simulink model "CryoDetFP"  (R2015b)
settings: Solver=ode45  SolverMode=SingleTasking  StartTime=0.0  StopTime=10e-5  MaxStep=1e-9  RelTol=1e-3
values from neighbouring files (symbols this model uses):
  Fclk = Fadc/2    (= 185000000)    [setupCryoFPGA.m]    (also in setupCryoNew.m)
  freqBusAddrBits = 4    [setupCryoNew.m]
  noise = ifft(exp(2i*pi*rand(1, noiseLen)) .* fft(fir1(noiseLen-1, noiseBW/Fclk*noiseSteps)))    [setupCryoFPGA.m]    (also in setupCryoNew.m = exp(2i*pi*rand(1, noiseLen)))
  noiseLen = 128    [setupCryoFPGA.m]    (also in setupCryoNew.m)
  noiseSteps = 32    [setupCryoFPGA.m]    (also in setupCryoNew.m)
  notch = tf( [1 a*wNotch/Q wNotch^2], [1 wNotch/Q wNotch^2])    [setupCryoNew.m]
  notch2 = tf( [1 a*wNotch/Q wNotch^2], [1 wNotch/Q wNotch^2])    [setupCryoNew.m]
  Tclk = 1/Fclk    (= 5.40540540541e-09)    [setupCryoFPGA.m]    (also in setupCryoNew.m)
undefined symbols (not defined in the file or in its folder): AXI4, Lite, notch3, notch4, xlipgetpartsetting
libraries: xbsIndex_r4 x1085
(part 3 of 8)

== system CryoDetFP/DspCore/AdcDac 0/twelveLineUDC 0 ==
  In1 : Inport
  BDC scope : Scope  NumInputPorts=2
  Constant : xbsIndex_r4/Constant  const=0  gui_display_data_type=Fixed-point  arith_type=Unsigned  n_bits=4  bin_pt=0  preci_type=Single  exp_width=8  frac_width=24  explicit_period=off  period=1  equ=P=C  opselect=C  inp2=PCIN>>17  opr=+  inp1=P  carry=CIN  dbl_ovrd=off  block_type=constant
  Constant1 : xbsIndex_r4/Constant  const=1  gui_display_data_type=Fixed-point  arith_type=Unsigned  n_bits=4  bin_pt=0  preci_type=Single  exp_width=8  frac_width=24  explicit_period=off  period=1  equ=P=C  opselect=C  inp2=PCIN>>17  opr=+  inp1=P  carry=CIN  dbl_ovrd=off  block_type=constant
  Constant10 : xbsIndex_r4/Constant  const=10  gui_display_data_type=Fixed-point  arith_type=Unsigned  n_bits=4  bin_pt=0  preci_type=Single  exp_width=8  frac_width=24  explicit_period=off  period=1  equ=P=C  opselect=C  inp2=PCIN>>17  opr=+  inp1=P  carry=CIN  dbl_ovrd=off  block_type=constant
  Constant11 : xbsIndex_r4/Constant  const=11  gui_display_data_type=Fixed-point  arith_type=Unsigned  n_bits=4  bin_pt=0  preci_type=Single  exp_width=8  frac_width=24  explicit_period=off  period=1  equ=P=C  opselect=C  inp2=PCIN>>17  opr=+  inp1=P  carry=CIN  dbl_ovrd=off  block_type=constant
  Constant12 : xbsIndex_r4/Constant  const=15  gui_display_data_type=Fixed-point  arith_type=Unsigned  n_bits=4  bin_pt=0  preci_type=Single  exp_width=8  frac_width=24  explicit_period=off  period=1  equ=P=C  opselect=C  inp2=PCIN>>17  opr=+  inp1=P  carry=CIN  dbl_ovrd=off  block_type=constant
  Constant2 : xbsIndex_r4/Constant  const=2  gui_display_data_type=Fixed-point  arith_type=Unsigned  n_bits=4  bin_pt=0  preci_type=Single  exp_width=8  frac_width=24  explicit_period=off  period=1  equ=P=C  opselect=C  inp2=PCIN>>17  opr=+  inp1=P  carry=CIN  dbl_ovrd=off  block_type=constant
  Constant3 : xbsIndex_r4/Constant  const=3  gui_display_data_type=Fixed-point  arith_type=Unsigned  n_bits=4  bin_pt=0  preci_type=Single  exp_width=8  frac_width=24  explicit_period=off  period=1  equ=P=C  opselect=C  inp2=PCIN>>17  opr=+  inp1=P  carry=CIN  dbl_ovrd=off  block_type=constant
  Constant4 : xbsIndex_r4/Constant  const=4  gui_display_data_type=Fixed-point  arith_type=Unsigned  n_bits=4  bin_pt=0  preci_type=Single  exp_width=8  frac_width=24  explicit_period=off  period=1  equ=P=C  opselect=C  inp2=PCIN>>17  opr=+  inp1=P  carry=CIN  dbl_ovrd=off  block_type=constant
  Constant5 : xbsIndex_r4/Constant  const=5  gui_display_data_type=Fixed-point  arith_type=Unsigned  n_bits=4  bin_pt=0  preci_type=Single  exp_width=8  frac_width=24  explicit_period=off  period=1  equ=P=C  opselect=C  inp2=PCIN>>17  opr=+  inp1=P  carry=CIN  dbl_ovrd=off  block_type=constant
  Constant6 : xbsIndex_r4/Constant  const=6  gui_display_data_type=Fixed-point  arith_type=Unsigned  n_bits=4  bin_pt=0  preci_type=Single  exp_width=8  frac_width=24  explicit_period=off  period=1  equ=P=C  opselect=C  inp2=PCIN>>17  opr=+  inp1=P  carry=CIN  dbl_ovrd=off  block_type=constant
  Constant7 : xbsIndex_r4/Constant  const=7  gui_display_data_type=Fixed-point  arith_type=Unsigned  n_bits=4  bin_pt=0  preci_type=Single  exp_width=8  frac_width=24  explicit_period=off  period=1  equ=P=C  opselect=C  inp2=PCIN>>17  opr=+  inp1=P  carry=CIN  dbl_ovrd=off  block_type=constant
  Constant8 : xbsIndex_r4/Constant  const=8  gui_display_data_type=Fixed-point  arith_type=Unsigned  n_bits=4  bin_pt=0  preci_type=Single  exp_width=8  frac_width=24  explicit_period=off  period=1  equ=P=C  opselect=C  inp2=PCIN>>17  opr=+  inp1=P  carry=CIN  dbl_ovrd=off  block_type=constant
  Constant9 : xbsIndex_r4/Constant  const=9  gui_display_data_type=Fixed-point  arith_type=Unsigned  n_bits=4  bin_pt=0  preci_type=Single  exp_width=8  frac_width=24  explicit_period=off  period=1  equ=P=C  opselect=C  inp2=PCIN>>17  opr=+  inp1=P  carry=CIN  dbl_ovrd=off  block_type=constant
  Counter : xbsIndex_r4/Counter  cnt_type=Count Limited  cnt_to=15  operation=Up  start_count=0  cnt_by_val=1  arith_type=Unsigned  n_bits=4  bin_pt=0  load_pin=off  rst=on  en=on  explicit_period=off  period=Tclk  use_behavioral_HDL=off  implementation=Fabric  dbl_ovrd=off  block_type=counter
  DAC Sum : Subsystem
  Delay : xbsIndex_r4/Delay  rst=off  infoeditControl=Selection of Reset will increase slice count due to use of real FFs and instead of SRLs  en=off  latency=6  reg_retiming=off  dbl_ovrd=off  block_type=delay
  Demux : Demux
  Gateway Out{1,7..10,23} (6 alike) : xbsIndex_r4/Gateway Out  inherit_from_input=off  hdl_port=off  rows=1  columns=1  UseAsDAC=off  DACChannel='1'  interface=None  automatic_assignment=on  address_offset=hex2dec('00')  intf_name=''  intf_description=''  timing_constraint=None  locs_specified=off  LOCs={}  io_standard={}  block_type=gatewayout
  Mux12X4 : Subsystem
  Mux6 : Mux  Inputs=2
  Mux7 : Mux  Inputs=2
  Relational : xbsIndex_r4/Relational  mode=a!=b  op_type=Bool  en=off  latency=0  dbl_ovrd=off  block_type=relational
  SBdemod : Subsystem
  Toolbar : xbsIndex_r4/Toolbar  func=xltoolbar  block_type=toolbar
      settings: infoedit=Toolbar
  oneLineUpDown0 : Subsystem
  oneLineUpDown1 : Subsystem
  oneLineUpDown10 : Subsystem
  oneLineUpDown11 : Subsystem
  oneLineUpDown2 : Subsystem
  oneLineUpDown3 : Subsystem
  oneLineUpDown4 : Subsystem
  oneLineUpDown5 : Subsystem
  oneLineUpDown6 : Subsystem
  oneLineUpDown7 : Subsystem
  oneLineUpDown8 : Subsystem
  oneLineUpDown9 : Subsystem
  synch scope : Scope  NumInputPorts=2
  toDAC : Outport
  demodulated : Outport  Port=2
  wires:
  [fpgaReset] -> Counter/1, Delay/1
  oneLineUpDown7/1(Out1) -> Mux12X4/8(line7)
  oneLineUpDown6/1(Out1) -> Mux12X4/7(line6)
  oneLineUpDown5/1(Out1) -> Mux12X4/6(line5)
  oneLineUpDown4/1(Out1) -> Mux12X4/5(line4)
  oneLineUpDown3/1(Out1) -> Mux12X4/4(line3)
  oneLineUpDown2/1(Out1) -> Mux12X4/3(line2)
  Mux12X4/1(Out1) -> SBdemod/1(In1)
  oneLineUpDown1/1(Out1) -> Mux12X4/2(line1)
  oneLineUpDown0/1(Out1) -> Mux12X4/1(line0)
  oneLineUpDown8/1(Out1) -> Mux12X4/9(line8)
  oneLineUpDown9/1(Out1) -> Mux12X4/10(line9)
  oneLineUpDown10/1(Out1) -> Mux12X4/11(line10)
  oneLineUpDown11/1(Out1) -> Mux12X4/12(line11)
  oneLineUpDown11/2(toDAC) -> DAC Sum/12(In12)
  oneLineUpDown10/2(toDAC) -> DAC Sum/11(In11)
  oneLineUpDown9/2(toDAC) -> DAC Sum/10(In10)
  oneLineUpDown8/2(toDAC) -> DAC Sum/9(In9)
  oneLineUpDown7/2(toDAC) -> DAC Sum/8(In8)
  oneLineUpDown6/2(toDAC) -> DAC Sum/7(In7)
  oneLineUpDown5/2(toDAC) -> DAC Sum/6(In6)
  oneLineUpDown4/2(toDAC) -> DAC Sum/5(In5)
  oneLineUpDown3/2(toDAC) -> DAC Sum/4(In4)
  oneLineUpDown2/2(toDAC) -> DAC Sum/3(In3)
  oneLineUpDown1/2(toDAC) -> DAC Sum/2(In2)
  oneLineUpDown0/2(toDAC) -> DAC Sum/1(In1)
  DAC Sum/1(Out1) -> toDAC/1
  SBdemod/1(AllComponents) -> demodulated/1
  Gateway Out10/1 -> Mux7/2
  Gateway Out9/1 -> Mux7/1
  Gateway Out8/1 -> Mux6/2
  Gateway Out7/1 -> Mux6/1
  Mux6/1 -> BDC scope/1
  Mux7/1 -> BDC scope/2
  Demux/1 -> Gateway Out7/1
  Demux/4 -> Gateway Out10/1
  Demux/3 -> Gateway Out9/1
  Demux/2 -> Gateway Out8/1
  Delay/1 -> Mux12X4/13(synch)
  Constant/1 -> oneLineUpDown0/2(addrIn)
  Constant1/1 -> oneLineUpDown1/2(addrIn)
  Constant2/1 -> oneLineUpDown2/2(addrIn)
  Constant3/1 -> oneLineUpDown3/2(addrIn)
  Constant4/1 -> oneLineUpDown4/2(addrIn)
  Constant5/1 -> oneLineUpDown5/2(addrIn)
  Constant6/1 -> oneLineUpDown6/2(addrIn)
  Constant7/1 -> oneLineUpDown7/2(addrIn)
  Constant8/1 -> oneLineUpDown8/2(addrIn)
  Constant9/1 -> oneLineUpDown9/2(addrIn)
  Constant10/1 -> oneLineUpDown10/2(addrIn)
  Constant11/1 -> oneLineUpDown11/2(addrIn)
  In1/1 -> oneLineUpDown6/1(In), oneLineUpDown8/1(In), oneLineUpDown9/1(In), oneLineUpDown10/1(In), oneLineUpDown11/1(In), oneLineUpDown7/1(In), Demux/1, oneLineUpDown5/1(In), oneLineUpDown4/1(In), oneLineUpDown3/1(In), oneLineUpDown2/1(In), oneLineUpDown1/1(In), oneLineUpDown0/1(In)
  Counter/1 -> Gateway Out23/1, Relational/2, oneLineUpDown2/3(synchIn), oneLineUpDown3/3(synchIn), oneLineUpDown4/3(synchIn), oneLineUpDown5/3(synchIn), oneLineUpDown6/3(synchIn), oneLineUpDown7/3(synchIn), oneLineUpDown8/3(synchIn), oneLineUpDown10/3(synchIn), oneLineUpDown11/3(synchIn), oneLineUpDown9/3(synchIn), oneLineUpDown1/3(synchIn), oneLineUpDown0/3(synchIn)
  Gateway Out23/1 -> synch scope/1
  Gateway Out1/1 -> synch scope/2
  Relational/1 -> Gateway Out1/1, Counter/2
  Constant12/1 -> Relational/1

== system CryoDetFP/DspCore/AdcDac 0/twelveLineUDC 1 ==
  note: Null for now, eventually copy twelveLineUDC 0
      | when we need more than 12 lines per ADC channel
  In1 : Inport
  Out1 : Outport
  wires:
  In1/1 -> Out1/1

== system CryoDetFP/DspCore/AdcDac 0/SBmodulator/Phase Modulator ==
  Iin : Inport
  Qin : Inport  Port=2
  Ipm : Inport  Port=3
  Qpm : Inport  Port=4
  AddSub : xbsIndex_r4/AddSub  mode=Subtraction  use_carryin=off  use_carryout=off  en=off  latency=1  precision=User Defined  arith_type="Signed  (2's comp)"  n_bits=16  bin_pt=15  quantization=Truncate  overflow=Wrap  use_behavioral_HDL=off  hw_selection=Fabric  pipelined=off  dbl_ovrd=off  block_type=addsub
  AddSub1 : xbsIndex_r4/AddSub  mode=Addition  use_carryin=off  use_carryout=off  en=off  latency=1  precision=User Defined  arith_type="Signed  (2's comp)"  n_bits=16  bin_pt=15  quantization=Truncate  overflow=Wrap  use_behavioral_HDL=off  hw_selection=Fabric  pipelined=off  dbl_ovrd=off  block_type=addsub
  Mult{1..4} (4 alike) : xbsIndex_r4/Mult  precision=User Defined  arith_type="Signed  (2's comp)"  n_bits=16  bin_pt=15  quantization=Truncate  overflow=Wrap  en=off  latency=3  use_behavioral_HDL=off  opt=Speed  use_embedded=on  optimum_pipeline=off  pipeline=on  dbl_ovrd=off  use_rpm=on  placement_style=Triangular  block_type=mult
  Iout : Outport
  Qout : Outport  Port=2
  wires:
  Iin/1 -> Mult4/1, Mult2/1
  Qin/1 -> Mult1/1, Mult3/1
  Ipm/1 -> Mult2/2, Mult1/2
  Qpm/1 -> Mult3/2, Mult4/2
  Mult2/1 -> AddSub/1
  Mult3/1 -> AddSub/2
  Mult1/1 -> AddSub1/1
  Mult4/1 -> AddSub1/2
  AddSub/1 -> Iout/1
  AddSub1/1 -> Qout/1

== system CryoDetFP/DspCore/AdcDac 0/dF/CplxProd ==
  tvalidIn : Inport
  Im_A : Inport  Port=2
  Re_A : Inport  Port=3
  Im_B : Inport  Port=4
  Re_B : Inport  Port=5
  AddSub : xbsIndex_r4/AddSub  mode=Subtraction  use_carryin=off  use_carryout=off  en=off  latency=3  precision=Full  arith_type=Unsigned  n_bits=16  bin_pt=14  quantization=Truncate  overflow=Wrap  use_behavioral_HDL=off  hw_selection=Fabric  pipelined=off  dbl_ovrd=off  block_type=addsub
  AddSub1 : xbsIndex_r4/AddSub  mode=Addition  use_carryin=off  use_carryout=off  en=off  latency=3  precision=Full  arith_type=Unsigned  n_bits=16  bin_pt=14  quantization=Truncate  overflow=Wrap  use_behavioral_HDL=off  hw_selection=Fabric  pipelined=off  dbl_ovrd=off  block_type=addsub
  Delay : xbsIndex_r4/Delay  rst=off  infoeditControl=Selection of Reset will increase slice count due to use of real FFs and instead of SRLs  en=off  latency=3  reg_retiming=off  dbl_ovrd=off  block_type=delay
  Delay1 : xbsIndex_r4/Delay  rst=off  infoeditControl=Selection of Reset will increase slice count due to use of real FFs and instead of SRLs  en=off  latency=3  reg_retiming=off  dbl_ovrd=off  block_type=delay
  Mult{,1..3} (4 alike) : xbsIndex_r4/Mult  precision=Full  arith_type="Signed  (2's comp)"  n_bits=16  bin_pt=14  quantization=Truncate  overflow=Wrap  en=off  latency=3  use_behavioral_HDL=off  opt=Speed  use_embedded=on  optimum_pipeline=off  pipeline=on  dbl_ovrd=off  use_rpm=on  placement_style=Triangular  block_type=mult
  tvalidOut : Outport
  Im_Out : Outport  Port=2
  Re_Out : Outport  Port=3
  wires:
  Delay/1 -> Delay1/1
  Mult2/1 -> AddSub1/1
  Mult/1 -> AddSub/1
  Mult1/1 -> AddSub/2
  Mult3/1 -> AddSub1/2
  Re_A/1 -> Mult3/1, Mult/1
  Im_A/1 -> Mult2/1, Mult1/1
  tvalidIn/1 -> Delay/1
  Im_B/1 -> Mult1/2, Mult3/2
  Re_B/1 -> Mult/2, Mult2/2
  Delay1/1 -> tvalidOut/1
  AddSub/1 -> Re_Out/1
  AddSub1/1 -> Im_Out/1

== system CryoDetFP/DspCore/AdcDac 0/dF/CplxProd1 ==
  tvalidIn : Inport
  Im_A : Inport  Port=2
  Re_A : Inport  Port=3
  Im_B : Inport  Port=4
  Re_B : Inport  Port=5
  AddSub : xbsIndex_r4/AddSub  mode=Subtraction  use_carryin=off  use_carryout=off  en=off  latency=3  precision=Full  arith_type=Unsigned  n_bits=16  bin_pt=14  quantization=Truncate  overflow=Wrap  use_behavioral_HDL=off  hw_selection=Fabric  pipelined=off  dbl_ovrd=off  block_type=addsub
  AddSub1 : xbsIndex_r4/AddSub  mode=Addition  use_carryin=off  use_carryout=off  en=off  latency=3  precision=Full  arith_type=Unsigned  n_bits=16  bin_pt=14  quantization=Truncate  overflow=Wrap  use_behavioral_HDL=off  hw_selection=Fabric  pipelined=off  dbl_ovrd=off  block_type=addsub
  Delay : xbsIndex_r4/Delay  rst=off  infoeditControl=Selection of Reset will increase slice count due to use of real FFs and instead of SRLs  en=off  latency=3  reg_retiming=off  dbl_ovrd=off  block_type=delay
  Delay1 : xbsIndex_r4/Delay  rst=off  infoeditControl=Selection of Reset will increase slice count due to use of real FFs and instead of SRLs  en=off  latency=3  reg_retiming=off  dbl_ovrd=off  block_type=delay
  Mult{,1..3} (4 alike) : xbsIndex_r4/Mult  precision=Full  arith_type="Signed  (2's comp)"  n_bits=16  bin_pt=14  quantization=Truncate  overflow=Wrap  en=off  latency=3  use_behavioral_HDL=off  opt=Speed  use_embedded=on  optimum_pipeline=off  pipeline=on  dbl_ovrd=off  use_rpm=on  placement_style=Triangular  block_type=mult
  tvalidOut : Outport
  Im_Out : Outport  Port=2
  Re_Out : Outport  Port=3
  wires:
  Delay/1 -> Delay1/1
  Mult2/1 -> AddSub1/1
  Mult/1 -> AddSub/1
  Mult1/1 -> AddSub/2
  Mult3/1 -> AddSub1/2
  Re_A/1 -> Mult3/1, Mult/1
  Im_A/1 -> Mult2/1, Mult1/1
  tvalidIn/1 -> Delay/1
  Im_B/1 -> Mult1/2, Mult3/2
  Re_B/1 -> Mult/2, Mult2/2
  Delay1/1 -> tvalidOut/1
  AddSub/1 -> Re_Out/1
  AddSub1/1 -> Im_Out/1

== system CryoDetFP/DspCore/AdcDac 0/dF/etaRAM ==
  note: 4 May 2016 Now floating point
  readAddr : Inport
  "etaBusIn " : Inport  Port=2
  Bus Selector : BusSelector  OutputSignals=channel,etaQ,etaI
  Concat : xbsIndex_r4/Concat  num_inputs=2  dbl_ovrd=off  block_type=concat
  Dual Port RAM : xbsIndex_r4/Dual Port RAM  depth=2^freqBusAddrBits  initVector=0  distributed_mem=Block RAM  init_a=0  init_b=0  rst_a=off  rst_b=off  en_a=off  en_b=off  latency=2  write_mode_A=Read Before Write  write_mode_B=Read After Write  optimize=Area  dbl_ovrd=off  block_type=dpram
  Gateway Out{1..3,13,26,29} (6 alike) : xbsIndex_r4/Gateway Out  inherit_from_input=off  hdl_port=off  rows=1  columns=1  UseAsDAC=off  DACChannel='1'  interface=None  automatic_assignment=on  address_offset=hex2dec('00')  intf_name=''  intf_description=''  timing_constraint=None  locs_specified=off  LOCs={}  io_standard={}  block_type=gatewayout
  Mux1 : Mux  Inputs=2
  Mux13 : Mux  Inputs=2
  Mux7 : Mux  Inputs=2
  Reinterpret : xbsIndex_r4/Reinterpret  force_arith_type=on  arith_type=Unsigned  force_bin_pt=on  bin_pt=0  block_type=reinterpret
  Reinterpret1 : xbsIndex_r4/Reinterpret  force_arith_type=on  arith_type=Unsigned  force_bin_pt=on  bin_pt=0  block_type=reinterpret
  Reinterpret2 : xbsIndex_r4/Reinterpret  force_arith_type=on  arith_type=Floating-point  force_bin_pt=on  bin_pt=24  block_type=reinterpret
  Reinterpret3 : xbsIndex_r4/Reinterpret  force_arith_type=on  arith_type=Floating-point  force_bin_pt=on  bin_pt=24  block_type=reinterpret
  Slice : xbsIndex_r4/Slice  nbits=32  boolean_output=off  mode=Upper Bit Location + Width  bit1=0  base1=MSB of Input  bit0=0  base0=LSB of Input  dbl_ovrd=off  block_type=slice
  Slice1 : xbsIndex_r4/Slice  nbits=32  boolean_output=off  mode=Lower Bit Location + Width  bit1=0  base1=MSB of Input  bit0=0  base0=LSB of Input  dbl_ovrd=off  block_type=slice
  Terminator3 : Terminator
  eta ram in out : Scope  NumInputPorts=3
  read : xbsIndex_r4/Constant  const=0  gui_display_data_type=Boolean  arith_type=Boolean  n_bits=16  bin_pt=14  preci_type=Single  exp_width=8  frac_width=24  explicit_period=off  period=1  equ=P=C  opselect=C  inp2=PCIN>>17  opr=+  inp1=P  carry=CIN  dbl_ovrd=off  block_type=constant
  write : xbsIndex_r4/Constant  const=1.0  gui_display_data_type=Boolean  arith_type=Boolean  n_bits=16  bin_pt=14  preci_type=Single  exp_width=8  frac_width=24  explicit_period=off  period=1  equ=P=C  opselect=C  inp2=PCIN>>17  opr=+  inp1=P  carry=CIN  dbl_ovrd=off  block_type=constant
  etaQ : Outport
  etaI : Outport  Port=2
  wires:
  read/1 -> Dual Port RAM/6
  Bus Selector/1 -> Gateway Out26/1, Dual Port RAM/1  "<channel>"
  write/1 -> Dual Port RAM/3
  Dual Port RAM/2 -> Slice1/1, Slice/1
  Dual Port RAM/1 -> Terminator3/1
  "etaBusIn "/1 -> Bus Selector/1
  Bus Selector/2 -> Gateway Out2/1, Reinterpret/1  "<etaQ>"
  Bus Selector/3 -> Gateway Out29/1, Reinterpret1/1  "<etaI>"
  Reinterpret1/1 -> Concat/2
  Reinterpret/1 -> Concat/1
  Concat/1 -> Dual Port RAM/2, Dual Port RAM/5
  Slice/1 -> Reinterpret2/1
  Slice1/1 -> Reinterpret3/1
  Reinterpret2/1 -> Gateway Out1/1, etaQ/1
  Reinterpret3/1 -> Gateway Out3/1, etaI/1
  Gateway Out29/1 -> Mux13/1
  Mux13/1 -> eta ram in out/2
  Gateway Out13/1 -> Mux7/2
  Gateway Out26/1 -> Mux7/1
  Mux7/1 -> eta ram in out/1
  Gateway Out2/1 -> Mux13/2
  readAddr/1 -> Gateway Out13/1, Dual Port RAM/4
  Gateway Out3/1 -> Mux1/1
  Mux1/1 -> eta ram in out/3
  Gateway Out1/1 -> Mux1/2

== system CryoDetFP/DspCore/AdcDac 0/eta/Complex Divide ==
  note: Complex multiplier has latency 6
  a_tvalid : Inport
  A_Q : Inport  Port=2
  A_I : Inport  Port=3
  b_tvalid : Inport  Port=4
  B_Q : Inport  Port=5
  B_I : Inport  Port=6
  AddSub : xbsIndex_r4/AddSub  mode=Addition  use_carryin=off  use_carryout=off  en=off  latency=3  precision=Full  arith_type="Signed  (2's comp)"  n_bits=48  bin_pt=44  quantization=Truncate  overflow=Flag as error  use_behavioral_HDL=on  hw_selection=Fabric  pipelined=off  dbl_ovrd=off  block_type=addsub
  CMult : xbsIndex_r4/CMult  const=-1  gui_display_data_type=Floating-point  const_n_bits=16  const_bin_pt=15  float_type=Single  exp_bits=8  fraction_bits=24  en=off  latency=1  precision=Full  arith_type="Signed  (2's comp)"  n_bits=32  bin_pt=30  quantization=Truncate  overflow=Wrap  use_behavioral_HDL=off  mem_type=Distributed RAM  pipeline=off  dbl_ovrd=off  block_type=cmult
  Constant : xbsIndex_r4/Constant  const=0  gui_display_data_type=Floating-point  arith_type=Floating-point  n_bits=63  bin_pt=15  preci_type=Single  exp_width=8  frac_width=24  explicit_period=off  period=1  equ=P=C  opselect=C  inp2=PCIN>>17  opr=+  inp1=P  carry=CIN  dbl_ovrd=off  block_type=constant
  Cplx Div 2 : Scope  NumInputPorts=3
  CplxProd : Subsystem
  Cpx Div : Scope  NumInputPorts=4
  Delay{,1..2,5} (4 alike) : xbsIndex_r4/Delay  rst=off  infoeditControl=Selection of Reset will increase slice count due to use of real FFs and instead of SRLs  en=off  latency=1  reg_retiming=on  dbl_ovrd=off  block_type=delay
  Delay3 : xbsIndex_r4/Delay  rst=off  infoeditControl=Selection of Reset will increase slice count due to use of real FFs and instead of SRLs  en=off  latency=8  reg_retiming=on  dbl_ovrd=off  block_type=delay
  Divide : xbsIndex_r4/Divide  flow_control=NonBlocking  axi_optimize_goal=Resources  algorithm_type=Radix2  infoedit1=Specify output fraction-width for Fixed-point division.  fractional_width=24  infoedit2=Specify latency for Floating-point division.  latency=8  rate=1  has_a_tlast=off  has_a_tuser=off  has_b_tlast=off  has_b_tuser=off  en=off  has_result_tready=off  result_tlast_behv=Pass_A_TLAST  has_underflow=on  has_overflow=on  has_invalid_op=on  has_divide_by_zero=on  fpo_op_type=mergeddivide  block_type=divide
      settings: infoedit=Blocking: Wait for data on all inputs, allow back-pressure.<br>NonBlocking: operate every cycle in which all inputs are valid, no back-pressure.
  Divide1 : xbsIndex_r4/Divide  flow_control=NonBlocking  axi_optimize_goal=Resources  algorithm_type=Radix2  infoedit1=Specify output fraction-width for Fixed-point division.  fractional_width=24  infoedit2=Specify latency for Floating-point division.  latency=8  rate=1  has_a_tlast=off  has_a_tuser=off  has_b_tlast=off  has_b_tuser=off  en=off  has_result_tready=off  result_tlast_behv=Pass_A_TLAST  has_underflow=on  has_overflow=on  has_invalid_op=on  has_divide_by_zero=on  fpo_op_type=mergeddivide  block_type=divide
      settings: infoedit=Blocking: Wait for data on all inputs, allow back-pressure.<br>NonBlocking: operate every cycle in which all inputs are valid, no back-pressure.
  Gateway Out{6..17} (12 alike) : xbsIndex_r4/Gateway Out  inherit_from_input=off  hdl_port=off  rows=1  columns=1  UseAsDAC=off  DACChannel='1'  interface=None  automatic_assignment=on  address_offset=hex2dec('00')  intf_name=''  intf_description=''  timing_constraint=None  locs_specified=off  LOCs={}  io_standard={}  block_type=gatewayout
  Mult : xbsIndex_r4/Mult  precision=Full  arith_type="Signed  (2's comp)"  n_bits=48  bin_pt=44  quantization=Truncate  overflow=Flag as error  en=off  latency=4  use_behavioral_HDL=on  opt=Speed  use_embedded=on  optimum_pipeline=on  pipeline=on  dbl_ovrd=off  use_rpm=on  placement_style=Triangular  block_type=mult
  Mult1 : xbsIndex_r4/Mult  precision=Full  arith_type="Signed  (2's comp)"  n_bits=48  bin_pt=44  quantization=Truncate  overflow=Flag as error  en=off  latency=4  use_behavioral_HDL=on  opt=Speed  use_embedded=on  optimum_pipeline=off  pipeline=on  dbl_ovrd=off  use_rpm=on  placement_style=Triangular  block_type=mult
  Mux{1,3..5,8..10} (7 alike) : Mux  Inputs=2
  Mux6 : xbsIndex_r4/Mux  inputs=2  en=off  latency=0  precision=Full  arith_type=Unsigned  n_bits=63  bin_pt=15  quantization=Truncate  overflow=Flag as error  dbl_ovrd=off  block_type=mux
  Mux7 : xbsIndex_r4/Mux  inputs=2  en=off  latency=0  precision=Full  arith_type=Unsigned  n_bits=63  bin_pt=15  quantization=Truncate  overflow=Flag as error  dbl_ovrd=off  block_type=mux
  Terminator5 : Terminator
  tvalidOut : Outport
  Out_Q : Outport  Port=2
  Out_I : Outport  Port=3
  invalid op : Outport  Port=4
  wires:
  a_tvalid/1 -> Gateway Out13/1, Gateway Out12/1, Delay/1
  A_Q/1 -> Delay1/1, Gateway Out14/1
  A_I/1 -> Delay2/1, Gateway Out15/1
  Divide/1 -> Mux7/2
  Mult1/1 -> AddSub/2
  AddSub/1 -> Divide/2, Divide1/2
  Divide1/4 -> Gateway Out11/1, invalid op/1, Mux6/1, Mux7/1
  Mux7/1 -> Gateway Out6/1, Out_Q/1
  Mux6/1 -> Out_I/1, Gateway Out7/1
  Mult/1 -> AddSub/1
  Gateway Out6/1 -> Mux3/1
  Gateway Out7/1 -> Mux3/2
  Gateway Out8/1 -> Mux4/1
  Gateway Out9/1 -> Mux4/2
  Gateway Out10/1 -> Mux5/1
  Gateway Out11/1 -> Mux5/2
  Divide1/1 -> Mux6/2
  Constant/1 -> Mux7/3, Mux6/3
  Delay5/1 -> CplxProd/5(Re_B)
  Delay2/1 -> CplxProd/3(Re_A)
  Delay1/1 -> CplxProd/2(Im_A)
  Delay/1 -> CplxProd/1(tvalidIn)
  B_Q/1 -> Mult1/1, Mult1/2, Gateway Out16/1, CMult/1
  B_I/1 -> Mult/1, Mult/2, Delay5/1, Gateway Out17/1
  CMult/1 -> CplxProd/4(Im_B)
  Gateway Out12/1 -> Mux8/1
  Gateway Out13/1 -> Mux8/2
  Gateway Out14/1 -> Mux9/1
  Gateway Out15/1 -> Mux9/2
  Gateway Out16/1 -> Mux10/1
  Gateway Out17/1 -> Mux10/2
  Mux8/1 -> Cplx Div 2/1
  Mux9/1 -> Cplx Div 2/2
  Mux10/1 -> Cplx Div 2/3
  b_tvalid/1 -> Terminator5/1
  CplxProd/2(Im_Out) -> Divide/1
  CplxProd/1(tvalidOut) -> Mux1/2, Delay3/1
  CplxProd/3(Re_Out) -> Divide1/1
  Divide1/2 -> Gateway Out8/1
  Divide1/3 -> Gateway Out9/1
  Divide1/5 -> Gateway Out10/1
  Mux3/1 -> Cpx Div/2
  Mux4/1 -> Cpx Div/3
  Mux5/1 -> Cpx Div/4
  Delay3/1 -> Mux1/1, tvalidOut/1
  Mux1/1 -> Cpx Div/1

== system CryoDetFP/DspCore/AdcDac 0/eta/CplxProd ==
  tvalidIn : Inport
  Im_A : Inport  Port=2
  Re_A : Inport  Port=3
  Im_B : Inport  Port=4
  Re_B : Inport  Port=5
  AddSub : xbsIndex_r4/AddSub  mode=Subtraction  use_carryin=off  use_carryout=off  en=off  latency=3  precision=Full  arith_type=Unsigned  n_bits=16  bin_pt=14  quantization=Truncate  overflow=Wrap  use_behavioral_HDL=off  hw_selection=Fabric  pipelined=off  dbl_ovrd=off  block_type=addsub
  AddSub1 : xbsIndex_r4/AddSub  mode=Addition  use_carryin=off  use_carryout=off  en=off  latency=3  precision=Full  arith_type=Unsigned  n_bits=16  bin_pt=14  quantization=Truncate  overflow=Wrap  use_behavioral_HDL=off  hw_selection=Fabric  pipelined=off  dbl_ovrd=off  block_type=addsub
  Delay : xbsIndex_r4/Delay  rst=off  infoeditControl=Selection of Reset will increase slice count due to use of real FFs and instead of SRLs  en=off  latency=3  reg_retiming=off  dbl_ovrd=off  block_type=delay
  Delay1 : xbsIndex_r4/Delay  rst=off  infoeditControl=Selection of Reset will increase slice count due to use of real FFs and instead of SRLs  en=off  latency=3  reg_retiming=off  dbl_ovrd=off  block_type=delay
  Mult{,1..3} (4 alike) : xbsIndex_r4/Mult  precision=Full  arith_type="Signed  (2's comp)"  n_bits=16  bin_pt=14  quantization=Truncate  overflow=Wrap  en=off  latency=3  use_behavioral_HDL=off  opt=Speed  use_embedded=on  optimum_pipeline=off  pipeline=on  dbl_ovrd=off  use_rpm=on  placement_style=Triangular  block_type=mult
  tvalidOut : Outport
  Im_Out : Outport  Port=2
  Re_Out : Outport  Port=3
  wires:
  Delay/1 -> Delay1/1
  Mult2/1 -> AddSub1/1
  Mult/1 -> AddSub/1
  Mult1/1 -> AddSub/2
  Mult3/1 -> AddSub1/2
  Re_A/1 -> Mult3/1, Mult/1
  Im_A/1 -> Mult2/1, Mult1/1
  tvalidIn/1 -> Delay/1
  Im_B/1 -> Mult1/2, Mult3/2
  Re_B/1 -> Mult/2, Mult2/2
  Delay1/1 -> tvalidOut/1
  AddSub/1 -> Re_Out/1
  AddSub1/1 -> Im_Out/1

== system CryoDetFP/DspCore/AdcDac 0/eta/CplxProd1 ==
  tvalidIn : Inport
  Im_A : Inport  Port=2
  Re_A : Inport  Port=3
  Im_B : Inport  Port=4
  Re_B : Inport  Port=5
  AddSub : xbsIndex_r4/AddSub  mode=Subtraction  use_carryin=off  use_carryout=off  en=off  latency=3  precision=Full  arith_type=Unsigned  n_bits=16  bin_pt=14  quantization=Truncate  overflow=Wrap  use_behavioral_HDL=off  hw_selection=Fabric  pipelined=off  dbl_ovrd=off  block_type=addsub
  AddSub1 : xbsIndex_r4/AddSub  mode=Addition  use_carryin=off  use_carryout=off  en=off  latency=3  precision=Full  arith_type=Unsigned  n_bits=16  bin_pt=14  quantization=Truncate  overflow=Wrap  use_behavioral_HDL=off  hw_selection=Fabric  pipelined=off  dbl_ovrd=off  block_type=addsub
  Delay : xbsIndex_r4/Delay  rst=off  infoeditControl=Selection of Reset will increase slice count due to use of real FFs and instead of SRLs  en=off  latency=3  reg_retiming=off  dbl_ovrd=off  block_type=delay
  Delay1 : xbsIndex_r4/Delay  rst=off  infoeditControl=Selection of Reset will increase slice count due to use of real FFs and instead of SRLs  en=off  latency=3  reg_retiming=off  dbl_ovrd=off  block_type=delay
  Mult{,1..3} (4 alike) : xbsIndex_r4/Mult  precision=Full  arith_type="Signed  (2's comp)"  n_bits=16  bin_pt=14  quantization=Truncate  overflow=Wrap  en=off  latency=3  use_behavioral_HDL=off  opt=Speed  use_embedded=on  optimum_pipeline=off  pipeline=on  dbl_ovrd=off  use_rpm=on  placement_style=Triangular  block_type=mult
  tvalidOut : Outport
  Im_Out : Outport  Port=2
  Re_Out : Outport  Port=3
  wires:
  Delay/1 -> Delay1/1
  Mult2/1 -> AddSub1/1
  Mult/1 -> AddSub/1
  Mult1/1 -> AddSub/2
  Mult3/1 -> AddSub1/2
  Re_A/1 -> Mult3/1, Mult/1
  Im_A/1 -> Mult2/1, Mult1/1
  tvalidIn/1 -> Delay/1
  Im_B/1 -> Mult1/2, Mult3/2
  Re_B/1 -> Mult/2, Mult2/2
  Delay1/1 -> tvalidOut/1
  AddSub/1 -> Re_Out/1
  AddSub1/1 -> Im_Out/1

== system CryoDetFP/DspCore/AdcDac 0/eta/CplxProd2 ==
  tvalidIn : Inport
  Im_A : Inport  Port=2
  Re_A : Inport  Port=3
  Im_B : Inport  Port=4
  Re_B : Inport  Port=5
  AddSub : xbsIndex_r4/AddSub  mode=Subtraction  use_carryin=off  use_carryout=off  en=off  latency=3  precision=Full  arith_type=Unsigned  n_bits=16  bin_pt=14  quantization=Truncate  overflow=Wrap  use_behavioral_HDL=off  hw_selection=Fabric  pipelined=off  dbl_ovrd=off  block_type=addsub
  AddSub1 : xbsIndex_r4/AddSub  mode=Addition  use_carryin=off  use_carryout=off  en=off  latency=3  precision=Full  arith_type=Unsigned  n_bits=16  bin_pt=14  quantization=Truncate  overflow=Wrap  use_behavioral_HDL=off  hw_selection=Fabric  pipelined=off  dbl_ovrd=off  block_type=addsub
  Delay : xbsIndex_r4/Delay  rst=off  infoeditControl=Selection of Reset will increase slice count due to use of real FFs and instead of SRLs  en=off  latency=3  reg_retiming=off  dbl_ovrd=off  block_type=delay
  Delay1 : xbsIndex_r4/Delay  rst=off  infoeditControl=Selection of Reset will increase slice count due to use of real FFs and instead of SRLs  en=off  latency=3  reg_retiming=off  dbl_ovrd=off  block_type=delay
  Mult{,1..3} (4 alike) : xbsIndex_r4/Mult  precision=Full  arith_type="Signed  (2's comp)"  n_bits=16  bin_pt=14  quantization=Truncate  overflow=Wrap  en=off  latency=3  use_behavioral_HDL=off  opt=Speed  use_embedded=on  optimum_pipeline=off  pipeline=on  dbl_ovrd=off  use_rpm=on  placement_style=Triangular  block_type=mult
  tvalidOut : Outport
  Im_Out : Outport  Port=2
  Re_Out : Outport  Port=3
  wires:
  Delay/1 -> Delay1/1
  Mult2/1 -> AddSub1/1
  Mult/1 -> AddSub/1
  Mult1/1 -> AddSub/2
  Mult3/1 -> AddSub1/2
  Re_A/1 -> Mult3/1, Mult/1
  Im_A/1 -> Mult2/1, Mult1/1
  tvalidIn/1 -> Delay/1
  Im_B/1 -> Mult1/2, Mult3/2
  Re_B/1 -> Mult/2, Mult2/2
  Delay1/1 -> tvalidOut/1
  AddSub/1 -> Re_Out/1
  AddSub1/1 -> Im_Out/1

== system CryoDetFP/DspCore/AdcDac 0/eta/LPF ==
  note: REF channel should not be low-passed!
      | Needs to have same bandwidth as signal channel
      | but latency must match
  note: streaming interface? so complex divide gets data at lower rate?
  note: tvalid
  note: Channel #
  note: Sig+
  note: Sig-
  note: Ref+
  note: Ref
  note: Sig
  note: Ref-
  In1 : Inport
  Bus Creator : BusCreator  Inputs=2
  Bus Creator1 : BusCreator  Inputs=2
  Bus Selector : BusSelector  OutputSignals=chanAndTvalid,signal2
  Bus Selector1 : BusSelector  OutputSignals=channel,valid
  Bus Selector2 : BusSelector  OutputSignals=channel,tvalid
  CIC Compiler 4.0 {1..10} (10 alike) : xbsIndex_r4/CIC Compiler 4.0   filter_type=Decimation  number_of_stages=3  differential_delay=1  number_of_channels=12  sample_rate_changes=Fixed  fixed_or_initial_rate=8  minimum_rate=8  maximum_rate=8  ratespecification=Sample_Period  sampleperiod=1  hardwareoversamplingrate=1  quantization=Truncation  output_data_width=24  use_xtreme_dsp_slice=off  use_streaming_interface=on  has_aclken=off  has_aresetn=on  has_dout_tready=off  trim_axipin_name=on  gui_behaviour=Sysgen_GUI  input_data_width=18  ip_name=CIC Compiler  ip_version=4.0  dsptool_ready=true  wrapper_available=true  port_translation_map={ 'aclken' => 'en', 'aresetn' => 'rst' }  ipcore_xco_need_fpga_part=true  ipcore_verbose=false  block_type=cic_compiler_v4_0
  CIC LPF Scope : Scope  NumInputPorts=6
  CIC LPF input scope : Scope  NumInputPorts=5
  CIC reset : Subsystem
  Constant4 : xbsIndex_r4/Constant  const=10  gui_display_data_type=Fixed-point  arith_type=Unsigned  n_bits=4  bin_pt=0  preci_type=Single  exp_width=8  frac_width=24  explicit_period=off  period=1  equ=P=C  opselect=C  inp2=PCIN>>17  opr=+  inp1=P  carry=CIN  dbl_ovrd=off  block_type=constant
  Demux{,3..6} (5 alike) : Demux  Outputs=2
  Demux1 : Demux  Outputs=6
  Display : Display
  Gateway Out{,1,5..18} (16 alike) : xbsIndex_r4/Gateway Out  inherit_from_input=off  hdl_port=off  rows=1  columns=1  UseAsDAC=off  DACChannel='1'  interface=None  automatic_assignment=on  address_offset=hex2dec('00')  intf_name=''  intf_description=''  timing_constraint=None  locs_specified=off  LOCs={}  io_standard={}  block_type=gatewayout
  LPF chan output : Scope  NumInputPorts=2
  Mux : Mux  Inputs=2
  Mux1 : Mux  Inputs=10
  Mux3 : Mux  Inputs=2
  Mux4 : Mux  Inputs=2
  Scale{,1..9} (10 alike) : xbsIndex_r4/Scale  scale_factor=-9  dbl_ovrd=off  block_type=scale
  Terminator : Terminator
  Out1 : Outport
  wires:
  Demux1/1 -> Terminator/1
  Demux1/2 -> Demux/1
  Demux1/3 -> Demux3/1
  Demux1/5 -> Demux5/1
  Demux1/6 -> Demux6/1
  Bus Selector/2 -> Demux1/1  "<signal2>"
  In1/1 -> Bus Selector/1
  Demux1/4 -> Demux4/1
  Demux/1 -> Gateway Out16/1, CIC Compiler 4.0 3/2
  Demux/2 -> CIC Compiler 4.0 1/2
  Demux3/1 -> CIC Compiler 4.0 2/2
  Demux3/2 -> CIC Compiler 4.0 4/2
  Demux5/1 -> CIC Compiler 4.0 7/2
  Demux5/2 -> CIC Compiler 4.0 8/2
  Demux6/1 -> CIC Compiler 4.0 9/2
  Demux6/2 -> CIC Compiler 4.0 10/2
  Bus Selector1/2 -> CIC Compiler 4.0 3/1, CIC Compiler 4.0 1/1, CIC Compiler 4.0 2/1, CIC Compiler 4.0 4/1, CIC Compiler 4.0 5/1, CIC Compiler 4.0 6/1, CIC Compiler 4.0 7/1, CIC Compiler 4.0 8/1, CIC Compiler 4.0 9/1, CIC Compiler 4.0 10/1  "<valid>"
  Bus Selector1/1 -> Gateway Out15/1, CIC reset/2(Channel), [ChanIn]  "<channel>"
  Bus Selector/1 -> Bus Selector1/1  "<chanAndTvalid>"
  CIC Compiler 4.0 3/3 -> Scale/1
  CIC Compiler 4.0 1/3 -> Scale1/1
  CIC Compiler 4.0 2/3 -> Scale2/1
  CIC Compiler 4.0 4/3 -> Scale3/1
  Demux4/1 -> CIC Compiler 4.0 5/2
  Demux4/2 -> CIC Compiler 4.0 6/2
  CIC Compiler 4.0 7/3 -> Scale4/1
  CIC Compiler 4.0 8/3 -> Scale5/1
  CIC Compiler 4.0 9/3 -> Scale6/1
  CIC Compiler 4.0 10/3 -> Scale7/1
  Mux1/1 -> Bus Creator/2
  Bus Creator/1 -> Out1/1
  Bus Creator1/1 -> Bus Creator/1, Bus Selector2/1
  Scale/1 -> Gateway Out1/1, Mux1/1
  Scale1/1 -> Mux1/2
  Scale2/1 -> Mux1/3
  Scale3/1 -> Mux1/4
  Scale4/1 -> Mux1/7
  Scale5/1 -> Mux1/8
  Scale6/1 -> Mux1/9
  Scale7/1 -> Mux1/10
  CIC Compiler 4.0 7/2 -> Bus Creator1/2  "tvalid"
  Scale8/1 -> Mux1/5
  Scale9/1 -> Mux1/6
  CIC Compiler 4.0 4/6 -> Gateway Out/1
  CIC Compiler 4.0 7/6 -> Bus Creator1/1  "channel"
  CIC Compiler 4.0 3/1 -> Gateway Out5/1
  CIC Compiler 4.0 3/2 -> Gateway Out6/1
  CIC Compiler 4.0 3/4 -> Gateway Out7/1
  CIC Compiler 4.0 3/5 -> Gateway Out8/1
  CIC Compiler 4.0 3/6 -> Gateway Out9/1
  CIC Compiler 4.0 3/7 -> Gateway Out10/1
  CIC Compiler 4.0 3/8 -> Gateway Out11/1
  Gateway Out11/1 -> Mux3/2
  Gateway Out10/1 -> Mux3/1
  Mux3/1 -> CIC LPF Scope/6
  Gateway Out9/1 -> CIC LPF Scope/5
  Gateway Out8/1 -> CIC LPF Scope/4
  Gateway Out7/1 -> CIC LPF Scope/3
  Gateway Out6/1 -> CIC LPF Scope/2
  CIC reset/1(notResetOut) -> Gateway Out18/1, CIC Compiler 4.0 3/4, CIC Compiler 4.0 1/4, CIC Compiler 4.0 2/4, CIC Compiler 4.0 4/4, CIC Compiler 4.0 5/4, CIC Compiler 4.0 6/4, CIC Compiler 4.0 7/4, CIC Compiler 4.0 8/4, CIC Compiler 4.0 9/4, CIC Compiler 4.0 10/4
  Constant4/1 -> CIC reset/3(N-2)
  [fpgaReset] -> Gateway Out14/1, CIC reset/1(resetIn)
  CIC reset/2(tlast) -> CIC Compiler 4.0 2/3, CIC Compiler 4.0 5/3, CIC Compiler 4.0 6/3, CIC Compiler 4.0 8/3, CIC Compiler 4.0 9/3, CIC Compiler 4.0 10/3, CIC Compiler 4.0 7/3, CIC Compiler 4.0 4/3, CIC Compiler 4.0 3/3, Gateway Out17/1, CIC Compiler 4.0 1/3
  Gateway Out18/1 -> CIC LPF input scope/5
  Gateway Out17/1 -> CIC LPF input scope/4
  Gateway Out16/1 -> CIC LPF input scope/3
  Gateway Out15/1 -> CIC LPF input scope/2
  Gateway Out14/1 -> CIC LPF input scope/1
  Gateway Out5/1 -> Mux4/2
  Gateway Out1/1 -> Mux4/1
  Mux4/1 -> CIC LPF Scope/1
  Bus Selector2/2 -> Gateway Out13/1  "<tvalid>"
  Bus Selector2/1 -> Gateway Out12/1  "<channel>"
  Gateway Out12/1 -> Mux/1
  Gateway Out13/1 -> Mux/2
  Mux/1 -> LPF chan output/1
  Gateway Out/1 -> LPF chan output/2, Display/1
  CIC Compiler 4.0 5/3 -> Scale8/1
  CIC Compiler 4.0 6/3 -> Scale9/1

== system CryoDetFP/DspCore/AdcDac 0/loopFilter/initial Frequencies ==
  note: Channel 15 used for none of above
  note: initial Frequencies
  note: select initial frequency
      | for now just mux from input registers
      | eventually configure RAM and loading protocol
  channel : Inport
  Gateway Out12 : xbsIndex_r4/Gateway Out  inherit_from_input=off  hdl_port=off  rows=1  columns=1  UseAsDAC=off  DACChannel='1'  interface=None  automatic_assignment=on  address_offset=hex2dec('00')  intf_name=''  intf_description=''  timing_constraint=None  locs_specified=off  LOCs={}  io_standard={}  block_type=gatewayout
  Gateway Out13 : xbsIndex_r4/Gateway Out  inherit_from_input=off  hdl_port=off  rows=1  columns=1  UseAsDAC=off  DACChannel='1'  interface=None  automatic_assignment=on  address_offset=hex2dec('00')  intf_name=''  intf_description=''  timing_constraint=None  locs_specified=off  LOCs={}  io_standard={}  block_type=gatewayout
  Mux : xbsIndex_r4/Mux  inputs=16  en=off  latency=0  precision=Full  arith_type=Unsigned  n_bits=24  bin_pt=24  quantization=Truncate  overflow=Wrap  dbl_ovrd=off  block_type=mux
  initial Freqs : Scope  NumInputPorts=2
  Fi : Outport
  wires:
  channel/1 -> Gateway Out12/1, Mux/1
  [F0] -> Mux/2
  [F1] -> Mux/3
  [F2] -> Mux/4
  [F3] -> Mux/5
  [F4] -> Mux/6
  [F5] -> Mux/7
  [F6] -> Mux/8
  [F7] -> Mux/9
  [F8] -> Mux/10
  [F9] -> Mux/11
  [F10] -> Mux/12
  [F11] -> Mux/14, Mux/15, Mux/16, Mux/17, Mux/13
  Mux/1 -> Gateway Out13/1, Fi/1
  Gateway Out13/1 -> initial Freqs/2
  Gateway Out12/1 -> initial Freqs/1

== system CryoDetFP/DspCore/AdcDac 0/twelveLineUDC 0/DAC Sum ==
  note: Final adder stages reduce to 16 bits
  note: DAC1 (odd samples)
  note: DAC0 (even samples)
  In1 : Inport
  In2 : Inport  Port=2
  In3 : Inport  Port=3
  In4 : Inport  Port=4
  In5 : Inport  Port=5
  In6 : Inport  Port=6
  In7 : Inport  Port=7
  In8 : Inport  Port=8
  In9 : Inport  Port=9
  In10 : Inport  Port=10
  In11 : Inport  Port=11
  In12 : Inport  Port=12
  AddSub{,1..19} (20 alike) : xbsIndex_r4/AddSub  mode=Addition  use_carryin=off  use_carryout=off  en=off  latency=3  precision=User Defined  arith_type="Signed  (2's comp)"  n_bits=20  bin_pt=15  quantization=Truncate  overflow=Wrap  use_behavioral_HDL=off  hw_selection=Fabric  pipelined=off  dbl_ovrd=off  block_type=addsub
  AddSub20 : xbsIndex_r4/AddSub  mode=Addition  use_carryin=off  use_carryout=off  en=off  latency=3  precision=User Defined  arith_type="Signed  (2's comp)"  n_bits=16  bin_pt=15  quantization="Round  (unbiased: +/- Inf)"  overflow=Saturate  use_behavioral_HDL=off  hw_selection=Fabric  pipelined=off  dbl_ovrd=off  block_type=addsub
  AddSub21 : xbsIndex_r4/AddSub  mode=Addition  use_carryin=off  use_carryout=off  en=off  latency=3  precision=User Defined  arith_type="Signed  (2's comp)"  n_bits=16  bin_pt=15  quantization="Round  (unbiased: +/- Inf)"  overflow=Saturate  use_behavioral_HDL=off  hw_selection=Fabric  pipelined=off  dbl_ovrd=off  block_type=addsub
  DAC sum scope : Scope  NumInputPorts=2
  DAC sum scope1 : Scope  NumInputPorts=6
  Demux{,1..11} (12 alike) : Demux  Outputs=2
  Gateway Out{,1..9} (10 alike) : xbsIndex_r4/Gateway Out  inherit_from_input=off  hdl_port=off  rows=1  columns=1  UseAsDAC=off  DACChannel='1'  interface=None  automatic_assignment=on  address_offset=hex2dec('00')  intf_name=''  intf_description=''  timing_constraint=None  locs_specified=off  LOCs={}  io_standard={}  block_type=gatewayout
  Mux : Mux  Inputs=2
  Mux1 : Mux  Inputs=2
  Mux2 : Mux  Inputs=2
  Out1 : Outport
  wires:
  In1/1 -> Demux1/1
  In2/1 -> Demux/1
  In3/1 -> Demux2/1
  In4/1 -> Demux3/1
  In5/1 -> Demux4/1
  In6/1 -> Demux5/1
  In7/1 -> Demux6/1
  In8/1 -> Demux7/1
  In9/1 -> Demux8/1
  In10/1 -> Demux9/1
  In11/1 -> Demux10/1
  Demux/1 -> Gateway Out5/1, AddSub/2
  Demux2/1 -> Gateway Out6/1, AddSub2/1
  Demux3/1 -> Gateway Out7/1, AddSub2/2
  Demux4/1 -> Gateway Out8/1, AddSub4/1
  Demux5/1 -> Gateway Out9/1, AddSub4/2
  Demux6/1 -> AddSub6/1
  Demux8/1 -> AddSub8/1
  In12/1 -> Demux11/1
  AddSub20/1 -> Mux/1
  AddSub21/1 -> Mux/2
  Mux/1 -> Out1/1
  Demux7/1 -> AddSub6/2
  Demux9/1 -> AddSub8/2
  Demux10/1 -> AddSub10/1
  Demux11/1 -> AddSub10/2
  Demux/2 -> AddSub1/1
  Demux1/2 -> AddSub1/2
  Demux11/2 -> AddSub11/1
  Demux10/2 -> AddSub11/2
  Demux9/2 -> AddSub9/1
  Demux8/2 -> AddSub9/2
  Demux7/2 -> AddSub7/1
  Demux6/2 -> AddSub7/2
  Demux5/2 -> AddSub5/1
  Demux4/2 -> AddSub5/2
  Demux3/2 -> AddSub3/1
  Demux2/2 -> AddSub3/2
  AddSub/1 -> AddSub12/1
  AddSub2/1 -> AddSub12/2
  AddSub4/1 -> AddSub13/1
  AddSub6/1 -> AddSub13/2
  AddSub8/1 -> AddSub14/1
  AddSub10/1 -> AddSub14/2
  AddSub12/1 -> AddSub15/1
  AddSub13/1 -> AddSub15/2
  AddSub15/1 -> AddSub20/1, Gateway Out/1
  AddSub14/1 -> Gateway Out1/1, AddSub20/2
  AddSub1/1 -> AddSub16/1
  AddSub3/1 -> AddSub16/2
  AddSub5/1 -> AddSub17/1
  AddSub7/1 -> AddSub17/2
  AddSub9/1 -> AddSub18/1
  AddSub11/1 -> AddSub18/2
  AddSub16/1 -> AddSub19/1
  AddSub17/1 -> AddSub19/2
  AddSub19/1 -> Gateway Out2/1, AddSub21/1
  AddSub18/1 -> AddSub21/2, Gateway Out3/1
  Gateway Out3/1 -> Mux2/2
  Gateway Out2/1 -> Mux2/1
  Gateway Out1/1 -> Mux1/2
  Gateway Out/1 -> Mux1/1
  Mux1/1 -> DAC sum scope/1
  Mux2/1 -> DAC sum scope/2
  Gateway Out4/1 -> DAC sum scope1/1
  Gateway Out5/1 -> DAC sum scope1/2
  Gateway Out6/1 -> DAC sum scope1/3
  Gateway Out7/1 -> DAC sum scope1/4
  Gateway Out8/1 -> DAC sum scope1/5
  Gateway Out9/1 -> DAC sum scope1/6
  Demux1/1 -> Gateway Out4/1, AddSub/1

== system CryoDetFP/DspCore/AdcDac 0/twelveLineUDC 0/Mux12X4 ==
  note: I think this will select a channel 1 or 2 ticks after it has updated,
      | which should work fine. But optimal would be to delay synch in by 11 ticks = N-1
  note: Channel ID
  note: Reference Q&I
  note: Signal Q&I
  note: Twelve busses 4-wide each time-division multiplexed onto a 4-wide bus
  line0 : Inport
  line1 : Inport  Port=2
  line2 : Inport  Port=3
  line3 : Inport  Port=4
  line4 : Inport  Port=5
  line5 : Inport  Port=6
  line6 : Inport  Port=7
  line7 : Inport  Port=8
  line8 : Inport  Port=9
  line9 : Inport  Port=10
  line10 : Inport  Port=11
  line11 : Inport  Port=12
  synch : Inport  Port=13
  "12x4 Mux out scope " : Scope  NumInputPorts=3
  Bus Creator : BusCreator  Inputs=2
  Counter : xbsIndex_r4/Counter  cnt_type=Count Limited  cnt_to=11  operation=Up  start_count=0  cnt_by_val=1  arith_type=Unsigned  n_bits=4  bin_pt=0  load_pin=off  rst=on  en=off  explicit_period=off  period=Tclk  use_behavioral_HDL=off  implementation=Fabric  dbl_ovrd=off  block_type=counter
  Delay1 : xbsIndex_r4/Delay  rst=off  infoeditControl=Selection of Reset will increase slice count due to use of real FFs and instead of SRLs  en=off  latency=1  reg_retiming=off  dbl_ovrd=off  block_type=delay
  Demux{,1..11} (12 alike) : Demux
  Gateway Out{1..8} (8 alike) : xbsIndex_r4/Gateway Out  inherit_from_input=off  hdl_port=off  rows=1  columns=1  UseAsDAC=off  DACChannel='1'  interface=None  automatic_assignment=on  address_offset=hex2dec('00')  intf_name=''  intf_description=''  timing_constraint=None  locs_specified=off  LOCs={}  io_standard={}  block_type=gatewayout
  Mux{,1..3} (4 alike) : xbsIndex_r4/Mux  inputs=12  en=off  latency=1  precision=Full  arith_type=Unsigned  n_bits=16  bin_pt=14  quantization=Truncate  overflow=Wrap  dbl_ovrd=off  block_type=mux
  Mux{4..9} (6 alike) : Mux  Inputs=2
  debug synch Scope : Scope  NumInputPorts=2
  Out1 : Outport
  wires:
  line0/1 -> Demux/1
  line5/1 -> Demux6/1
  line4/1 -> Demux5/1
  line3/1 -> Demux4/1
  line2/1 -> Demux3/1
  line1/1 -> Demux1/1
  Demux/1 -> Gateway Out4/1, Mux/2
  Demux/2 -> Mux1/2
  Demux/3 -> Mux2/2
  Demux/4 -> Mux3/2
  Demux1/1 -> Mux/3
  Demux1/2 -> Mux1/3
  Demux1/3 -> Mux2/3
  Demux1/4 -> Mux3/3
  Demux3/1 -> Mux/4
  Demux3/2 -> Mux1/4
  Demux3/3 -> Mux2/4
  Demux3/4 -> Mux3/4
  line11/1 -> Demux11/1
  line10/1 -> Demux10/1
  line9/1 -> Demux9/1
  line8/1 -> Demux8/1
  line7/1 -> Demux7/1
  line6/1 -> Demux2/1
  Demux4/1 -> Mux/5
  Demux4/2 -> Mux1/5
  Demux4/3 -> Mux2/5
  Demux4/4 -> Mux3/5
  Demux5/1 -> Mux/6
  Demux5/2 -> Mux1/6
  Demux5/3 -> Mux2/6
  Demux5/4 -> Mux3/6
  Demux6/1 -> Mux/7
  Demux6/2 -> Mux1/7
  Demux6/3 -> Mux2/7
  Demux6/4 -> Mux3/7
  Demux2/1 -> Mux/8
  Demux2/3 -> Mux2/8
  Demux2/4 -> Mux3/8
  Demux7/1 -> Mux/9
  Demux7/2 -> Mux1/9
  Demux2/2 -> Mux1/8
  Demux7/3 -> Mux2/9
  Demux7/4 -> Mux3/9
  Demux8/1 -> Mux/10
  Demux8/2 -> Mux1/10
  Demux8/3 -> Mux2/10
  Demux8/4 -> Mux3/10
  Demux9/1 -> Mux/11
  Demux9/2 -> Mux1/11
  Demux9/3 -> Mux2/11
  Demux9/4 -> Mux3/11
  Demux10/1 -> Mux/12
  Demux10/2 -> Mux1/12
  Demux10/3 -> Mux2/12
  Demux10/4 -> Mux3/12
  Demux11/1 -> Mux/13
  Demux11/2 -> Mux1/13
  Demux11/3 -> Mux2/13
  Demux11/4 -> Mux3/13
  synch/1 -> Gateway Out8/1, Counter/1
  Mux/1 -> Gateway Out2/1, Mux6/1
  Mux1/1 -> Gateway Out3/1, Mux6/2
  Mux2/1 -> Gateway Out6/1, Mux5/1
  Mux3/1 -> Gateway Out7/1, Mux5/2
  Mux6/1 -> Mux4/1
  Mux5/1 -> Mux4/2
  Counter/1 -> Mux2/1, Delay1/1, Mux1/1, Mux3/1, Mux/1, Gateway Out5/1
  Mux4/1 -> Bus Creator/2
  Delay1/1 -> Gateway Out1/1, Bus Creator/1  "channel"
  Bus Creator/1 -> Out1/1
  Gateway Out7/1 -> Mux7/2
  Gateway Out6/1 -> Mux7/1
  Gateway Out3/1 -> Mux8/2
  Gateway Out2/1 -> Mux8/1
  Mux7/1 -> "12x4 Mux out scope "/3
  Mux8/1 -> "12x4 Mux out scope "/2
  Gateway Out1/1 -> "12x4 Mux out scope "/1
  Gateway Out8/1 -> debug synch Scope/2
  Gateway Out4/1 -> Mux9/2
  Mux9/1 -> debug synch Scope/1
  Gateway Out5/1 -> Mux9/1
